simulink model "speed_control_rotativo_open_loop"  (R2022b)
settings: Solver=VariableStepAuto  StartTime=0.0  StopTime=10  FixedStep=0.00001  MaxStep=0.0001  RelTol=1e-3
libraries: simulink x4, autolibim x1, mcbplantlib x1, mcbcontrolslib x1
settings Model: Creator=mique  LastModifiedBy=mique
settings SolverCC: ZeroCrossAlgorithm=Adaptive
settings DebuggingCC: IgnoredZcDiagnostic=none

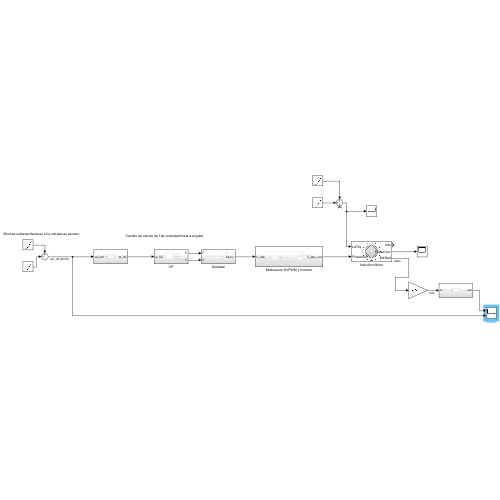
[thumbnail: Simulink's stored preview of the top-level diagram]
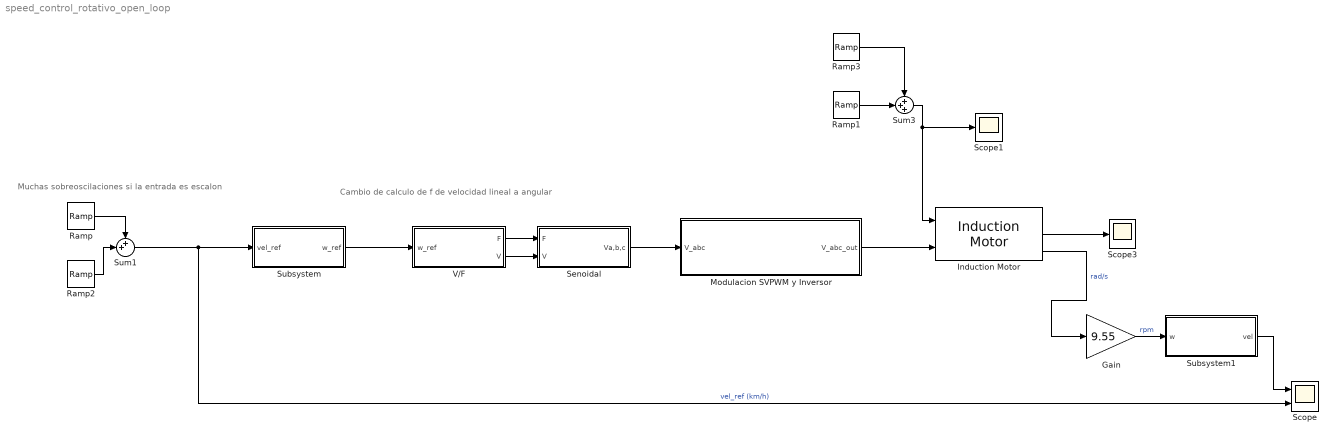
== system speed_control_rotativo_open_loop ==
  note: Cambio de calculo de f de velocidad lineal a angular
  note: Muchas sobreoscilaciones si la entrada es escalon
  Gain : Gain  Gain=9.55
  Induction Motor : autolibim/Induction Motor  sim_type=Continuous  Ts=0.001  port_config=Torque  P=2  Zs=[1.77 0.0139]  Zr="[1.34  0.0121]"  Lm=0.3687  mechanical=[0.01 0.059 0.01]  theta_init=0  omega_init=0  RefBlkName='autolibim/Induction Motor'  aMode=5
      settings: LibrarySourceBlock=mcblib/Electrical Systems/Motors/Induction Motor
  Modulacion SVPWM y Inversor : Subsystem
  Ramp : simulink/Sources/Ramp  slope=-5  start=7  InitialOutput=0
  Ramp1 : simulink/Sources/Ramp  slope=0.5  start=0.1  InitialOutput=0
  Ramp2 : simulink/Sources/Ramp  slope=5  start=0  InitialOutput=0
  Ramp3 : simulink/Sources/Ramp  slope=-0.5  start=5  InitialOutput=0
  Scope : Scope  NumInputPorts=2
  Scope1 : Scope
  Scope3 : Scope
  Senoidal : Subsystem
  Subsystem : Subsystem
  Subsystem1 : Subsystem
  Sum1 : Sum  Inputs=++|
  Sum3 : Sum  Inputs=+++
  V/F : Subsystem
  wires:
  V/F/1(F) -> Senoidal/1(F)
  Induction Motor/2 -> Scope3/1
  V/F/2(V) -> Senoidal/2(V)
  Induction Motor/3 -> Gain/1  "rad/s"
  Ramp/1 -> Sum1/1
  Ramp2/1 -> Sum1/2
  Ramp1/1 -> Sum3/2
  Ramp3/1 -> Sum3/1
  Subsystem/1(w_ref) -> V/F/1(w_ref)
  Gain/1 -> Subsystem1/1(w)  "rpm"
  Subsystem1/1(vel) -> Scope/1
  Senoidal/1(Va,b,c) -> Modulacion SVPWM y Inversor/1(V_abc)
  Modulacion SVPWM y Inversor/1(V_abc_out) -> Induction Motor/2
  Sum1/1 -> Scope/2, Subsystem/1(vel_ref)  "vel_ref (km/h)"
  Sum3/1 -> Scope1/1, Induction Motor/1

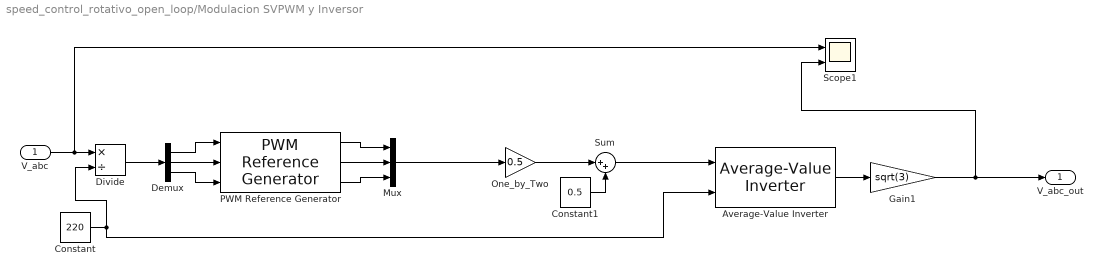
== system speed_control_rotativo_open_loop/Modulacion SVPWM y Inversor ==
  V_abc : Inport
  Average-Value Inverter : mcbplantlib/Average-Value Inverter
      settings: LibrarySourceBlock=mcblib/Electrical Systems/Inverters/Average-Value Inverter
  Constant : Constant  Value=220
  Constant1 : Constant  Value=0.5  SampleTime=-1
  Demux : Demux  Outputs=3
  Divide : Product  Inputs=*/
  Gain1 : Gain  Gain=sqrt(3)
  Mux : Mux  Inputs=3
  One_by_Two : Gain  Gain=0.5  RndMeth=Simplest  OutDataTypeStr=Inherit: Same as input
  PWM Reference Generator : mcbcontrolslib/PWM Reference Generator  inSignal=Vabc  modType=SVM: space vector modulation
      settings: LibrarySourceBlock=mcbhdllib/Controls/Math Transforms/PWM Reference Generator
  Scope1 : Scope  NumInputPorts=2
  Sum : Sum  Inputs=|++
  V_abc_out : Outport
  wires:
  V_abc/1 -> Scope1/1, Divide/1
  PWM Reference Generator/1 -> Mux/1
  Demux/3 -> PWM Reference Generator/3
  Gain1/1 -> V_abc_out/1, Scope1/2
  Mux/1 -> One_by_Two/1
  PWM Reference Generator/2 -> Mux/2
  Constant/1 -> Divide/2, Average-Value Inverter/2
  Sum/1 -> Average-Value Inverter/1
  Demux/2 -> PWM Reference Generator/2
  PWM Reference Generator/3 -> Mux/3
  Demux/1 -> PWM Reference Generator/1
  One_by_Two/1 -> Sum/1
  Constant1/1 -> Sum/2
  Divide/1 -> Demux/1
  Average-Value Inverter/1 -> Gain1/1

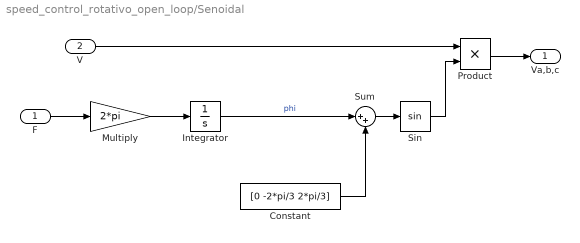
== system speed_control_rotativo_open_loop/Senoidal ==
  F : Inport
  V : Inport  Port=2
  Constant : Constant  Value=[0 -2*pi/3 2*pi/3]
  Integrator : Integrator  WrapState=on
  Multiply : Gain  Gain=2*pi
  Product : Product
  Sin : Trigonometry
  Sum : Sum  Inputs=|++
  Va,b,c : Outport
  wires:
  Integrator/1 -> Sum/1  "phi"
  Constant/1 -> Sum/2
  Sum/1 -> Sin/1
  V/1 -> Product/1
  Sin/1 -> Product/2
  Product/1 -> Va,b,c/1
  F/1 -> Multiply/1
  Multiply/1 -> Integrator/1

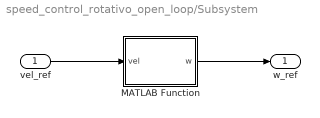
== system speed_control_rotativo_open_loop/Subsystem ==
  vel_ref : Inport
  MATLAB Function : MATLAB Function  TreatAsAtomicUnit=on
  w_ref : Outport
  wires:
  vel_ref/1 -> MATLAB Function/1(vel)
  MATLAB Function/1(w) -> w_ref/1

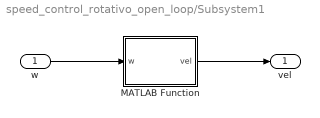
== system speed_control_rotativo_open_loop/Subsystem1 ==
  w : Inport
  MATLAB Function : MATLAB Function  TreatAsAtomicUnit=on
  vel : Outport
  wires:
  w/1 -> MATLAB Function/1(w)
  MATLAB Function/1(vel) -> vel/1

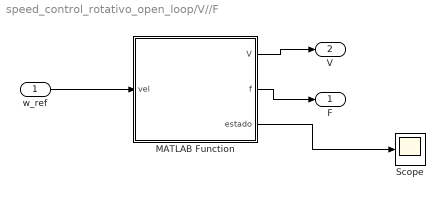
== system speed_control_rotativo_open_loop/V//F ==
  w_ref : Inport
  MATLAB Function : MATLAB Function  TreatAsAtomicUnit=on
  Scope : Scope
  F : Outport
  V : Outport  Port=2
  wires:
  w_ref/1 -> MATLAB Function/1(vel)
  MATLAB Function/1(V) -> V/1
  MATLAB Function/2(f) -> F/1
  MATLAB Function/3(estado) -> Scope/1

== matlab function speed_control_rotativo_open_loop/Subsystem/MATLAB Function ==
  data: vel input; w output
function w = fcn(vel)

%Paso polar en metros
paso_polar=0.114;
%De km/h a m/s
vel_m=vel/3.6;

num_parejas_Polos=6;


distancia_angular_parejas_polos=2*pi/(num_parejas_Polos*2);


w=vel_m/paso_polar*distancia_angular_parejas_polos;

== matlab function speed_control_rotativo_open_loop/V//F/MATLAB Function ==
  data: vel input; V output; f output; estado output
function [V,f,estado]= v_f(vel)
estado=0;
num_parejas_Polos=2;

%Velocidad en RPM
f=vel*num_parejas_Polos/60;

if(f==0)
    f=0.0001;
    V=0;
    return
end

%F en HZ

%Comprobar valores
f_corte_inf=1;
V_min=30;
V_max=220;
f_corte_sup=f_corte_inf*V_max/V_min;

if(f<f_corte_inf)
    V=V_min;
    estado=0;
elseif(f<f_corte_sup)
    V=V_min/f_corte_inf*f;
    estado=1;
else
    V=V_max;
    estado=2;
end

== matlab function speed_control_rotativo_open_loop/Subsystem1/MATLAB Function ==
  data: w input; vel output
function vel = fcn(w)

%Paso polar en metros
paso_polar=0.114;

num_parejas_Polos=6;

distancia_angular_parejas_polos=2*pi/(num_parejas_Polos*2);


vel_m=w*paso_polar/distancia_angular_parejas_polos;

%De m/s a km/h
vel=vel_m*3.6;
